simulink model "d3_model_FixedPointFilter_byhand"  (R2020a)
settings: Solver=ode45  StartTime=0.0  StopTime=Inf  RelTol=1e-3  EnableMultiTasking=on
libraries: dspsnks4 x1, dspvision x1
settings Model: ModifiedByFormat=The MathWorks Inc.  Creator=The MathWorks, Inc.  LastModifiedBy=The MathWorks Inc.
settings DataIOCC: LimitDataPoints=on  SaveFormat=Array  ReturnWorkspaceOutputs=off  SignalLoggingName=logsOut
settings OptimizationCC: ExpressionDepthLimit=2147483647  InitFltsAndDblsToZero=on  EfficientMapNaN2IntZero=off  LifeSpan=inf
settings DebuggingCC: UnderspecifiedInitializationDetection=Classic  MergeDetectMultiDrivingBlocksExec=none  SignalResolutionControl=TryResolveAllWithWarning  MultiTaskDSMMsg=warning  MultiTaskCondExecSysMsg=none  ParameterPrecisionLossMsg=none  FcnCallInpInsideContextMsg=warning  StateNameClashWarn=warning  SFUnexpectedBacktrackingDiag=warning  SFNoUnconditionalDefaultTransitionDiag=warning  SFExecutionAtInitializationDiag=none  ArithmeticOperatorsInVariantConditions=warning
settings HardwareCC: ProdBitPerPointer=32  ProdBitPerSizeT=32  ProdBitPerPtrDiffT=32  ProdLargestAtomicFloat=None  ProdIntDivRoundTo=Undefined  ProdEndianess=Unspecified  ProdWordSize=32  ProdHWDeviceType=Specified
settings ModelReferenceCC: PropagateSignalLabelsOutOfModel=off
settings SFSimCC: SimUseLocalCustomCode=off  CustomCodeUndefinedFunction=UseInterfaceOnly
settings RTWCC: RTWUseLocalCustomCode=off
settings CodeAppCC: StateflowObjectComments=on
settings GRTTargetCC: TargetFcnLib=ansi_tfl_tmw_new.mat  TargetLangStandard=C89/C90 (ANSI)  CombineOutputUpdateFcns=off  GRTInterface=on
settings ConfigComp: CovMetricSettings=dw  CovHtmlReporting=on  CovSaveCumulativeToWorkspaceVar=on  CovSaveSingleToWorkspaceVar=on  CovExternalEMLEnable=off  CovSFcnEnable=off

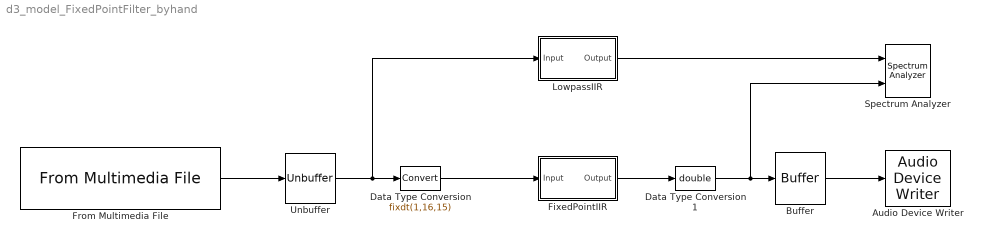
== system d3_model_FixedPointFilter_byhand ==
  Audio Device Writer : dspsnks4/Audio Device Writer  Driver=DirectSound  Device=Default  InheritSampleRate=on  SampleRate=8000  BitDepth=16-bit integer  BufferSize=4096  NumBuffers=10  DefaultOutputChannelMapping=on  OutputChannelMapping=1:2  OutputNumUnderrunSamples=off  DriverIdx=1  DeviceWarnFlag=''
  Buffer : Buffer  N=1024  OutputFrames=off
  Data Type Conversion : DataTypeConversion  OutDataTypeStr=fixdt(1,16,15)
  Data Type Conversion1 : DataTypeConversion  OutDataTypeStr=double
  FixedPointIIR : Subsystem  Tag=FilterWizardSubSystem
      settings: ErrorFcn=dspFilterRealizedInBasicElemsAlgLoopErrFcnCallback
  From Multimedia File : dspvision/From Multimedia File  inputFilename=mix.mp3  readRange=[1 Inf]  loop=on  numPlays=inf  outputStreams=Audio only  videoDataType=single  audioDataType=double  inheritSampleTime=on  userDefinedSampleTime=1/30  noAudioOutput=off  isIntensityVideo=off  fourcc=RGB  colorVideoFormat=Separate color signals  outputEOF=off  dataOrg=Column-major  audioFrameSize=1024  computeAudioFrameSize=off  outSamplingMode=Sample based
  LowpassIIR : Subsystem  Tag=FilterWizardSubSystem
      settings: ErrorFcn=dspFilterRealizedInBasicElemsAlgLoopErrFcnCallback
  Spectrum Analyzer : SpectrumAnalyzer  NumInputPorts=2
  Unbuffer : Unbuffer
  wires:
  FixedPointIIR/1(Output) -> Data Type Conversion1/1
  From Multimedia File/1 -> Unbuffer/1
  Unbuffer/1 -> LowpassIIR/1(Input), Data Type Conversion/1
  Buffer/1 -> Audio Device Writer/1
  Data Type Conversion/1 -> FixedPointIIR/1(Input)
  Data Type Conversion1/1 -> Spectrum Analyzer/2, Buffer/1
  LowpassIIR/1(Output) -> Spectrum Analyzer/1

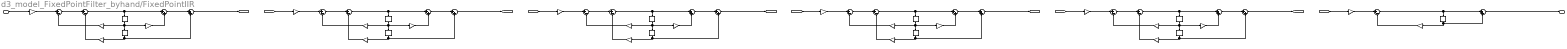
== system d3_model_FixedPointFilter_byhand/FixedPointIIR ==
  Input : Inport
  Delay{11..16,21..25} (11 alike) : Delay  DelayLength=1  InitialCondition=0
  SumA{21..26,31..35} (11 alike) : Sum  Inputs=|+-  RndMeth=Nearest  SaturateOnIntegerOverflow=on  OutDataTypeStr=Inherit: Same as first input
  SumB{21..26,31..35} (11 alike) : Sum  Inputs=|++  RndMeth=Nearest  SaturateOnIntegerOverflow=on  OutDataTypeStr=Inherit: Same as first input
  a(2)(1) : Gain  Gain=-1.87887411164094287  ParamDataTypeStr=double  RndMeth=Nearest  SaturateOnIntegerOverflow=on  OutDataTypeStr=Inherit: Same as input
  a(2)(2) : Gain  Gain=-1.86938889660215057  ParamDataTypeStr=double  RndMeth=Nearest  SaturateOnIntegerOverflow=on  OutDataTypeStr=Inherit: Same as input
  a(2)(3) : Gain  Gain=-1.85103857272687655  ParamDataTypeStr=double  RndMeth=Nearest  SaturateOnIntegerOverflow=on  OutDataTypeStr=Inherit: Same as input
  a(2)(4) : Gain  Gain=-1.81356044973371122  ParamDataTypeStr=double  RndMeth=Nearest  SaturateOnIntegerOverflow=on  OutDataTypeStr=Inherit: Same as input
  a(2)(5) : Gain  Gain=-1.75714642696634749  ParamDataTypeStr=double  RndMeth=Nearest  SaturateOnIntegerOverflow=on  OutDataTypeStr=Inherit: Same as input
  a(2)(6) : Gain  Gain=-0.862147885429035199  ParamDataTypeStr=double  RndMeth=Nearest  SaturateOnIntegerOverflow=on  OutDataTypeStr=Inherit: Same as input
  a(3)(1) : Gain  Gain=0.995334312073497873  ParamDataTypeStr=double  RndMeth=Nearest  SaturateOnIntegerOverflow=on  OutDataTypeStr=Inherit: Same as input
  a(3)(2) : Gain  Gain=0.981652820727124231  ParamDataTypeStr=double  RndMeth=Nearest  SaturateOnIntegerOverflow=on  OutDataTypeStr=Inherit: Same as input
  a(3)(3) : Gain  Gain=0.952110814082869572  ParamDataTypeStr=double  RndMeth=Nearest  SaturateOnIntegerOverflow=on  OutDataTypeStr=Inherit: Same as input
  a(3)(4) : Gain  Gain=0.89052601668852216  ParamDataTypeStr=double  RndMeth=Nearest  SaturateOnIntegerOverflow=on  OutDataTypeStr=Inherit: Same as input
  a(3)(5) : Gain  Gain=0.797502108834443613  ParamDataTypeStr=double  RndMeth=Nearest  SaturateOnIntegerOverflow=on  OutDataTypeStr=Inherit: Same as input
  b(2)(1) : Gain  Gain=-1.87466164839833538  ParamDataTypeStr=double  RndMeth=Nearest  SaturateOnIntegerOverflow=on  OutDataTypeStr=Inherit: Same as input
  b(2)(2) : Gain  Gain=-1.86921829081474966  ParamDataTypeStr=double  RndMeth=Nearest  SaturateOnIntegerOverflow=on  OutDataTypeStr=Inherit: Same as input
  b(2)(3) : Gain  Gain=-1.85135145393246603  ParamDataTypeStr=double  RndMeth=Nearest  SaturateOnIntegerOverflow=on  OutDataTypeStr=Inherit: Same as input
  b(2)(4) : Gain  Gain=-1.79039300454486972  ParamDataTypeStr=double  RndMeth=Nearest  SaturateOnIntegerOverflow=on  OutDataTypeStr=Inherit: Same as input
  b(2)(5) : Gain  Gain=-1.46966101911981695  ParamDataTypeStr=double  RndMeth=Nearest  SaturateOnIntegerOverflow=on  OutDataTypeStr=Inherit: Same as input
  s(1) : Gain  Gain=0.398391035946394134  ParamDataTypeStr=double  RndMeth=Nearest  SaturateOnIntegerOverflow=on  OutDataTypeStr=Inherit: Same as input
  s(2) : Gain  Gain=0.858406919624770004  ParamDataTypeStr=double  RndMeth=Nearest  SaturateOnIntegerOverflow=on  OutDataTypeStr=Inherit: Same as input
  s(3) : Gain  Gain=0.679941001979759818  ParamDataTypeStr=double  RndMeth=Nearest  SaturateOnIntegerOverflow=on  OutDataTypeStr=Inherit: Same as input
  s(4) : Gain  Gain=0.367189877359255124  ParamDataTypeStr=double  RndMeth=Nearest  SaturateOnIntegerOverflow=on  OutDataTypeStr=Inherit: Same as input
  s(5) : Gain  Gain=0.0760941271960040994  ParamDataTypeStr=double  RndMeth=Nearest  SaturateOnIntegerOverflow=on  OutDataTypeStr=Inherit: Same as input
  s(6) : Gain  Gain=0.160756089508545807  ParamDataTypeStr=double  RndMeth=Nearest  SaturateOnIntegerOverflow=on  OutDataTypeStr=Inherit: Same as input
  Output : Outport
  wires:
  Delay16/1 -> SumB26/2, a(2)(6)/1
  a(2)(6)/1 -> SumA26/2
  SumB26/1 -> Output/1
  SumA26/1 -> Delay16/1, SumB26/1
  s(6)/1 -> SumA26/1
  [Sect5] -> s(6)/1
  Delay25/1 -> SumB35/2, a(3)(5)/1
  a(3)(5)/1 -> SumA35/2
  b(2)(5)/1 -> SumB25/2
  Delay15/1 -> Delay25/1, b(2)(5)/1, a(2)(5)/1
  a(2)(5)/1 -> SumA25/2
  SumB35/1 -> [Sect5]
  SumB25/1 -> SumB35/1
  SumA35/1 -> Delay15/1, SumB25/1
  SumA25/1 -> SumA35/1
  s(5)/1 -> SumA25/1
  [Sect4] -> s(5)/1
  Delay24/1 -> SumB34/2, a(3)(4)/1
  a(3)(4)/1 -> SumA34/2
  b(2)(4)/1 -> SumB24/2
  Delay14/1 -> Delay24/1, b(2)(4)/1, a(2)(4)/1
  a(2)(4)/1 -> SumA24/2
  SumB34/1 -> [Sect4]
  SumB24/1 -> SumB34/1
  SumA34/1 -> Delay14/1, SumB24/1
  SumA24/1 -> SumA34/1
  s(4)/1 -> SumA24/1
  [Sect3] -> s(4)/1
  Delay23/1 -> SumB33/2, a(3)(3)/1
  a(3)(3)/1 -> SumA33/2
  b(2)(3)/1 -> SumB23/2
  Delay13/1 -> Delay23/1, b(2)(3)/1, a(2)(3)/1
  a(2)(3)/1 -> SumA23/2
  SumB33/1 -> [Sect3]
  SumB23/1 -> SumB33/1
  SumA33/1 -> Delay13/1, SumB23/1
  SumA23/1 -> SumA33/1
  s(3)/1 -> SumA23/1
  [Sect2] -> s(3)/1
  Delay22/1 -> SumB32/2, a(3)(2)/1
  a(3)(2)/1 -> SumA32/2
  b(2)(2)/1 -> SumB22/2
  Delay12/1 -> Delay22/1, b(2)(2)/1, a(2)(2)/1
  a(2)(2)/1 -> SumA22/2
  SumB32/1 -> [Sect2]
  SumB22/1 -> SumB32/1
  SumA32/1 -> Delay12/1, SumB22/1
  SumA22/1 -> SumA32/1
  s(2)/1 -> SumA22/1
  [Sect1] -> s(2)/1
  Delay21/1 -> SumB31/2, a(3)(1)/1
  a(3)(1)/1 -> SumA31/2
  b(2)(1)/1 -> SumB21/2
  Delay11/1 -> Delay21/1, b(2)(1)/1, a(2)(1)/1
  a(2)(1)/1 -> SumA21/2
  SumB31/1 -> [Sect1]
  SumB21/1 -> SumB31/1
  SumA31/1 -> Delay11/1, SumB21/1
  SumA21/1 -> SumA31/1
  s(1)/1 -> SumA21/1
  Input/1 -> s(1)/1

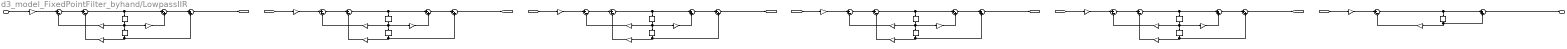
== system d3_model_FixedPointFilter_byhand/LowpassIIR ==
  Input : Inport
  Delay{11..16,21..25} (11 alike) : Delay  DelayLength=1  InitialCondition=0
  SumA{21..26,31..35} (11 alike) : Sum  Inputs=|+-  RndMeth=Nearest  SaturateOnIntegerOverflow=on  OutDataTypeStr=Inherit: Same as first input
  SumB{21..26,31..35} (11 alike) : Sum  Inputs=|++  RndMeth=Nearest  SaturateOnIntegerOverflow=on  OutDataTypeStr=Inherit: Same as first input
  a(2)(1) : Gain  Gain=-1.87887411164094287  ParamDataTypeStr=double  RndMeth=Nearest  SaturateOnIntegerOverflow=on  OutDataTypeStr=Inherit: Same as input
  a(2)(2) : Gain  Gain=-1.86938889660215057  ParamDataTypeStr=double  RndMeth=Nearest  SaturateOnIntegerOverflow=on  OutDataTypeStr=Inherit: Same as input
  a(2)(3) : Gain  Gain=-1.85103857272687655  ParamDataTypeStr=double  RndMeth=Nearest  SaturateOnIntegerOverflow=on  OutDataTypeStr=Inherit: Same as input
  a(2)(4) : Gain  Gain=-1.81356044973371122  ParamDataTypeStr=double  RndMeth=Nearest  SaturateOnIntegerOverflow=on  OutDataTypeStr=Inherit: Same as input
  a(2)(5) : Gain  Gain=-1.75714642696634749  ParamDataTypeStr=double  RndMeth=Nearest  SaturateOnIntegerOverflow=on  OutDataTypeStr=Inherit: Same as input
  a(2)(6) : Gain  Gain=-0.862147885429035199  ParamDataTypeStr=double  RndMeth=Nearest  SaturateOnIntegerOverflow=on  OutDataTypeStr=Inherit: Same as input
  a(3)(1) : Gain  Gain=0.995334312073497873  ParamDataTypeStr=double  RndMeth=Nearest  SaturateOnIntegerOverflow=on  OutDataTypeStr=Inherit: Same as input
  a(3)(2) : Gain  Gain=0.981652820727124231  ParamDataTypeStr=double  RndMeth=Nearest  SaturateOnIntegerOverflow=on  OutDataTypeStr=Inherit: Same as input
  a(3)(3) : Gain  Gain=0.952110814082869572  ParamDataTypeStr=double  RndMeth=Nearest  SaturateOnIntegerOverflow=on  OutDataTypeStr=Inherit: Same as input
  a(3)(4) : Gain  Gain=0.89052601668852216  ParamDataTypeStr=double  RndMeth=Nearest  SaturateOnIntegerOverflow=on  OutDataTypeStr=Inherit: Same as input
  a(3)(5) : Gain  Gain=0.797502108834443613  ParamDataTypeStr=double  RndMeth=Nearest  SaturateOnIntegerOverflow=on  OutDataTypeStr=Inherit: Same as input
  b(2)(1) : Gain  Gain=-1.87466164839833538  ParamDataTypeStr=double  RndMeth=Nearest  SaturateOnIntegerOverflow=on  OutDataTypeStr=Inherit: Same as input
  b(2)(2) : Gain  Gain=-1.86921829081474966  ParamDataTypeStr=double  RndMeth=Nearest  SaturateOnIntegerOverflow=on  OutDataTypeStr=Inherit: Same as input
  b(2)(3) : Gain  Gain=-1.85135145393246603  ParamDataTypeStr=double  RndMeth=Nearest  SaturateOnIntegerOverflow=on  OutDataTypeStr=Inherit: Same as input
  b(2)(4) : Gain  Gain=-1.79039300454486972  ParamDataTypeStr=double  RndMeth=Nearest  SaturateOnIntegerOverflow=on  OutDataTypeStr=Inherit: Same as input
  b(2)(5) : Gain  Gain=-1.46966101911981695  ParamDataTypeStr=double  RndMeth=Nearest  SaturateOnIntegerOverflow=on  OutDataTypeStr=Inherit: Same as input
  s(1) : Gain  Gain=0.398391035946394134  ParamDataTypeStr=double  RndMeth=Nearest  SaturateOnIntegerOverflow=on  OutDataTypeStr=Inherit: Same as input
  s(2) : Gain  Gain=0.858406919624770004  ParamDataTypeStr=double  RndMeth=Nearest  SaturateOnIntegerOverflow=on  OutDataTypeStr=Inherit: Same as input
  s(3) : Gain  Gain=0.679941001979759818  ParamDataTypeStr=double  RndMeth=Nearest  SaturateOnIntegerOverflow=on  OutDataTypeStr=Inherit: Same as input
  s(4) : Gain  Gain=0.367189877359255124  ParamDataTypeStr=double  RndMeth=Nearest  SaturateOnIntegerOverflow=on  OutDataTypeStr=Inherit: Same as input
  s(5) : Gain  Gain=0.0760941271960040994  ParamDataTypeStr=double  RndMeth=Nearest  SaturateOnIntegerOverflow=on  OutDataTypeStr=Inherit: Same as input
  s(6) : Gain  Gain=0.160756089508545807  ParamDataTypeStr=double  RndMeth=Nearest  SaturateOnIntegerOverflow=on  OutDataTypeStr=Inherit: Same as input
  Output : Outport
  wires:
  Input/1 -> s(1)/1
  s(1)/1 -> SumA21/1
  SumA21/1 -> SumA31/1
  SumA31/1 -> SumB21/1, Delay11/1
  SumB21/1 -> SumB31/1
  SumB31/1 -> [Sect1]
  a(2)(1)/1 -> SumA21/2
  Delay11/1 -> a(2)(1)/1, b(2)(1)/1, Delay21/1
  b(2)(1)/1 -> SumB21/2
  a(3)(1)/1 -> SumA31/2
  Delay21/1 -> a(3)(1)/1, SumB31/2
  [Sect1] -> s(2)/1
  s(2)/1 -> SumA22/1
  SumA22/1 -> SumA32/1
  SumA32/1 -> SumB22/1, Delay12/1
  SumB22/1 -> SumB32/1
  SumB32/1 -> [Sect2]
  a(2)(2)/1 -> SumA22/2
  Delay12/1 -> a(2)(2)/1, b(2)(2)/1, Delay22/1
  b(2)(2)/1 -> SumB22/2
  a(3)(2)/1 -> SumA32/2
  Delay22/1 -> a(3)(2)/1, SumB32/2
  [Sect2] -> s(3)/1
  s(3)/1 -> SumA23/1
  SumA23/1 -> SumA33/1
  SumA33/1 -> SumB23/1, Delay13/1
  SumB23/1 -> SumB33/1
  SumB33/1 -> [Sect3]
  a(2)(3)/1 -> SumA23/2
  Delay13/1 -> a(2)(3)/1, b(2)(3)/1, Delay23/1
  b(2)(3)/1 -> SumB23/2
  a(3)(3)/1 -> SumA33/2
  Delay23/1 -> a(3)(3)/1, SumB33/2
  [Sect3] -> s(4)/1
  s(4)/1 -> SumA24/1
  SumA24/1 -> SumA34/1
  SumA34/1 -> SumB24/1, Delay14/1
  SumB24/1 -> SumB34/1
  SumB34/1 -> [Sect4]
  a(2)(4)/1 -> SumA24/2
  Delay14/1 -> a(2)(4)/1, b(2)(4)/1, Delay24/1
  b(2)(4)/1 -> SumB24/2
  a(3)(4)/1 -> SumA34/2
  Delay24/1 -> a(3)(4)/1, SumB34/2
  [Sect4] -> s(5)/1
  s(5)/1 -> SumA25/1
  SumA25/1 -> SumA35/1
  SumA35/1 -> SumB25/1, Delay15/1
  SumB25/1 -> SumB35/1
  SumB35/1 -> [Sect5]
  a(2)(5)/1 -> SumA25/2
  Delay15/1 -> a(2)(5)/1, b(2)(5)/1, Delay25/1
  b(2)(5)/1 -> SumB25/2
  a(3)(5)/1 -> SumA35/2
  Delay25/1 -> a(3)(5)/1, SumB35/2
  [Sect5] -> s(6)/1
  s(6)/1 -> SumA26/1
  SumA26/1 -> SumB26/1, Delay16/1
  SumB26/1 -> Output/1
  a(2)(6)/1 -> SumA26/2
  Delay16/1 -> a(2)(6)/1, SumB26/2
